simulink model "generic_IsaacV3"  (R2015a)
settings: Solver=ode3  StartTime=0.0  StopTime=inf  FixedStep=0.001  RelTol=1e-3
values from neighbouring files (symbols this model uses):
  coast_domain = 0.1    [LoadVar.m]
  DifferentialFactor = 0.5    [LoadVar.m]
  g = 9.81    [LoadVar.m]
  GearRatio = 10.364    [LoadVar.m]
  Gr = 10.32    [LoadVar.m]
  Lf = 0.78    [LoadVar.m]
  Lr = 0.745    [LoadVar.m]
  M = 265    [LoadVar.m]
  max_coast_Nm = 0    [LoadVar.m]
  MaxSteeringAngle = 24.635    [LoadVar.m]
  mu_max = 1.5    [LoadVar.m]
  ped_max_limiet = 1    [LoadVar.m]
  pedal_position_maxacc = 0.9    [LoadVar.m]
  Reff = 0.2325    [LoadVar.m]
  regen_activation_kph = 15    [LoadVar.m]
  slewbreak_domain = 0.15    [LoadVar.m]
  Sr = 0.6    [LoadVar.m]
  T_max_Nm = 40    [LoadVar.m]
  T_min_Nm = -15    [LoadVar.m]
  TireRadius = 0.4572/2    (= 0.2286)    [LoadVar.m]
  Tmax = 40    [LoadVar.m]
  TrackLength = 1.534    [LoadVar.m]
  TrackWidth = 1.200    (= 1.2)    [LoadVar.m]
libraries: CarMaker4SL x21, simulink x7
(part 1 of 3)
settings Model: ExtModeAutoUpdateStatusClock=off  Creator=fh  LastModifiedBy=Alexander
settings DataIOCC: SignalLoggingSaveFormat=ModelDataLogs  SignalLoggingName=sigsOut
settings OptimizationCC: BooleanDataType=off  ExpressionDepthLimit=2147483647  InitFltsAndDblsToZero=on
settings DebuggingCC: SaveWithParameterizedLinksMsg=none  UnderspecifiedInitializationDetection=Classic  MergeDetectMultiDrivingBlocksExec=none  SignalResolutionControl=TryResolveAllWithWarning  MultiTaskDSMMsg=warning  MultiTaskCondExecSysMsg=none  FcnCallInpInsideContextMsg=UseLocalSettings  StateNameClashWarn=warning
settings HardwareCC: TargetLongLongMode=on  TargetIntDivRoundTo=Zero  TargetEndianess=LittleEndian  TargetHWDeviceType=MATLAB Host  ProdEqTarget=off
settings CodeAppCC: MaxIdLength=63
settings GRTTargetCC: TargetFcnLib=ansi_tfl_tmw.mat  CombineOutputUpdateFcns=off  GRTInterface=on

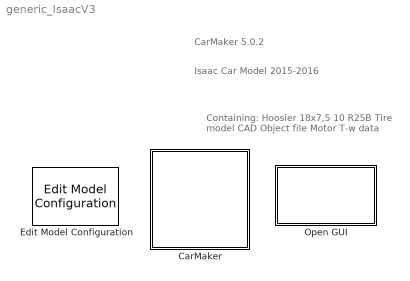
== system generic_IsaacV3 ==
  note: Isaac Car Model 2015-2016
  note: Containing:
      | Hoosier 18x7,5 10 R25B Tire model
      | CAD Object file
      | Motor T-w data
  note: CarMaker 5.0.2
  CarMaker : Subsystem  TreatAsAtomicUnit=on
      mask Display: image(imread('CarMaker4SLss.bmp'));
  Edit Model Configuration : CarMaker4SL/Edit Model Configuration
  Open GUI : Subsystem  LoadFcn=if ~length(which('cmcmd')), cmenv; end
      settings: OpenFcn=cmblockmagic('gui_fix_display'); CM_Simulink
      mask Display: image(imread('CarMakerGUI.bmp'));

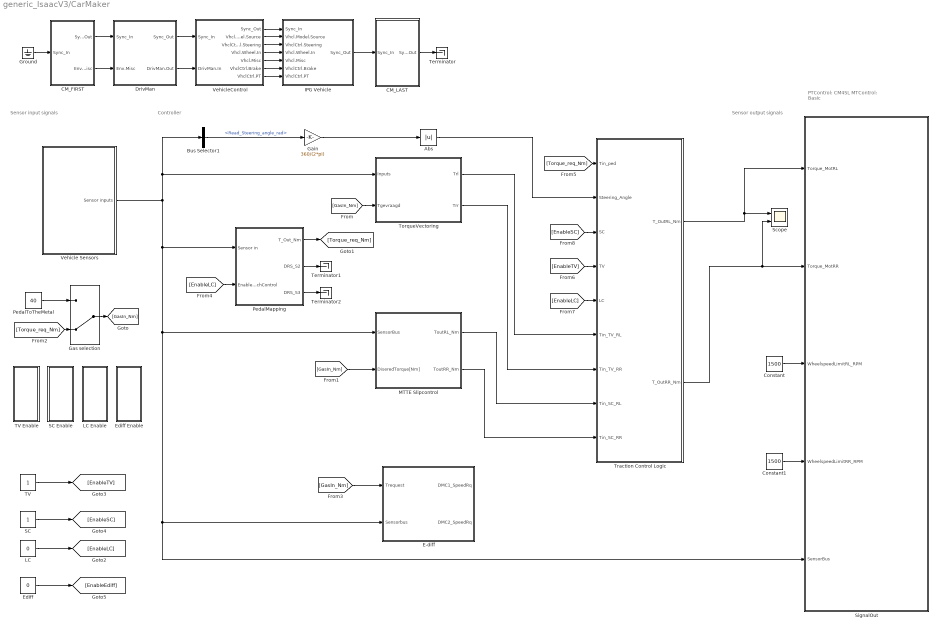
== system generic_IsaacV3/CarMaker ==
  note: PTControl: CM4SL
      | MTControl: Basic
  note: Controller
  note: Sensor output signals
  note: Sensor input signals
  Abs : Abs
  Bus Selector1 : BusSelector  OutputSignals=SensorBus.Read_Steering_angle_rad
  CM_FIRST : Subsystem
  CM_LAST : Subsystem
  Constant : Constant  Value=1500
  Constant1 : Constant  Value=1500
  DrivMan : Subsystem
  E-diff : Subsystem
  Ediff : Constant  Value=0
  Ediff Enable : Subsystem  DialogController=hmiCreateDDGDialog  IsWebBlock=on  mask(MathWorksWebBlock){webBlockId=a87a3f71-7ab5-45be-a85e-108e57319b55, webBlockType=toggleswitch, ShowInLibBrowser=on, ShowInitialText=on, HMISrcModelName=generic_IsaacV3}
      mask prompts: webBlockId "WebBlock Id"; webBlockType "WebBlock Type"; HMISrcModelName "Source Model"
      mask Help: helpview([docroot '/mapfiles/simulink.map'], 'hmi_toggle_switch')
      mask Display:
      | if strcmp(get_param(bdroot(gcb),'BlockDiagramType'), 'library')
      |     image([(matlabroot) '/toolbox/simulink/hmi/icons/ToggleSwitch.png']);
      | end
  Gain : Gain  Gain=360/(2*pi)
  Gas selection : ManualSwitch  CurrentSetting=0
  Ground : Ground
  IPG Vehicle : Subsystem  TreatAsAtomicUnit=on
  LC : Constant  Value=0
  LC Enable : Subsystem  DialogController=hmiCreateDDGDialog  IsWebBlock=on  mask(MathWorksWebBlock){webBlockId=f0719819-69bc-48b2-89e1-4e9d590658cc, webBlockType=toggleswitch, ShowInLibBrowser=on, ShowInitialText=on, HMISrcModelName=generic_IsaacV3}
      mask prompts: webBlockId "WebBlock Id"; webBlockType "WebBlock Type"; HMISrcModelName "Source Model"
      mask Help: helpview([docroot '/mapfiles/simulink.map'], 'hmi_toggle_switch')
      mask Display:
      | if strcmp(get_param(bdroot(gcb),'BlockDiagramType'), 'library')
      |     image([(matlabroot) '/toolbox/simulink/hmi/icons/ToggleSwitch.png']);
      | end
  MTTE Slipcontrol : Subsystem
  PedalMapping : Subsystem
  PedalToTheMetal : Constant  Value=40
  SC : Constant
  SC Enable : Subsystem  DialogController=hmiCreateDDGDialog  IsWebBlock=on  mask(MathWorksWebBlock){webBlockId=0a73dbf7-03b2-456b-97db-f8b49fcd234d, webBlockType=toggleswitch, ShowInLibBrowser=on, ShowInitialText=on, HMISrcModelName=generic_IsaacV3}
      mask prompts: webBlockId "WebBlock Id"; webBlockType "WebBlock Type"; HMISrcModelName "Source Model"
      mask Help: helpview([docroot '/mapfiles/simulink.map'], 'hmi_toggle_switch')
      mask Display:
      | if strcmp(get_param(bdroot(gcb),'BlockDiagramType'), 'library')
      |     image([(matlabroot) '/toolbox/simulink/hmi/icons/ToggleSwitch.png']);
      | end
  Scope : Scope  NumInputPorts=2
      settings: YMin=-20~-20  YMax=50~50  SaveName=ScopeData7
  SignalOut : Subsystem
  TV : Constant
  TV Enable : Subsystem  DialogController=hmiCreateDDGDialog  IsWebBlock=on  mask(MathWorksWebBlock){webBlockId=11ac5f76-cd76-4bde-b9bd-54c96ed035c7, webBlockType=toggleswitch, ShowInLibBrowser=on, ShowInitialText=on, HMISrcModelName=generic_IsaacV3}
      mask prompts: webBlockId "WebBlock Id"; webBlockType "WebBlock Type"; HMISrcModelName "Source Model"
      mask Help: helpview([docroot '/mapfiles/simulink.map'], 'hmi_toggle_switch')
      mask Display:
      | if strcmp(get_param(bdroot(gcb),'BlockDiagramType'), 'library')
      |     image([(matlabroot) '/toolbox/simulink/hmi/icons/ToggleSwitch.png']);
      | end
  Terminator : Terminator
  Terminator1 : Terminator
  Terminator2 : Terminator
  TorqueVectoring : Subsystem
  Traction Control Logic : Stateflow chart  TreatAsAtomicUnit=on
  Vehicle Sensors : Subsystem
  VehicleControl : Subsystem
  wires:
  DrivMan/2(DrivMan.Out) -> VehicleControl/2(DrivMan.In)
  DrivMan/1(Sync_Out) -> VehicleControl/1(Sync_In)
  CM_FIRST/2(Env.Misc) -> DrivMan/2(Env.Misc)
  CM_FIRST/1(Sync_Out) -> DrivMan/1(Sync_In)
  CM_LAST/1(Sync_Out) -> Terminator/1
  IPG Vehicle/1(Sync_Out) -> CM_LAST/1(Sync_In)
  VehicleControl/1(Sync_Out) -> IPG Vehicle/1(Sync_In)
  VehicleControl/3(VhclCtrl.Steering) -> IPG Vehicle/3(VhclCtrl.Steering)
  VehicleControl/4(Vhcl.Wheel.In) -> IPG Vehicle/4(Vhcl.Wheel.In)
  VehicleControl/5(Vhcl.Misc) -> IPG Vehicle/5(Vhcl.Misc)
  VehicleControl/6(VhclCtrl.Brake) -> IPG Vehicle/6(VhclCtrl.Brake)
  VehicleControl/7(VhclCtrl.PT) -> IPG Vehicle/7(VhclCtrl.PT)
  VehicleControl/2(Vhcl.Model.Source) -> IPG Vehicle/2(Vhcl.Model.Source)
  Ground/1 -> CM_FIRST/1(Sync_In)
  Vehicle Sensors/1(Sensor inputs) -> SignalOut/5(SensorBus), E-diff/2(Sensorbus), MTTE Slipcontrol/1(SensorBus), PedalMapping/1(Sensor in), Bus Selector1/1, TorqueVectoring/1(Inputs)
  PedalToTheMetal/1 -> Gas selection/1
  Gas selection/1 -> [GasIn_Nm]
  [GasIn_Nm] -> TorqueVectoring/2(Tgevraagd)
  [GasIn_Nm] -> MTTE Slipcontrol/2(DiseredTorque[Nm])
  PedalMapping/1(T_Out_Nm) -> [Torque_req_Nm]
  [Torque_req_Nm] -> Gas selection/2
  [GasIn_Nm] -> E-diff/1(Trequest)
  Constant/1 -> SignalOut/3(WheelspeedLimitRL_RPM)
  Constant1/1 -> SignalOut/4(WheelspeedLimitRR_RPM)
  [EnableLC] -> PedalMapping/2(EnableLaunchControl)
  LC/1 -> [EnableLC]
  TV/1 -> [EnableTV]
  SC/1 -> [EnableSC]
  Ediff/1 -> [EnableEdiff]
  Bus Selector1/1 -> Gain/1  "<Read_Steering_angle_rad>"
  Gain/1 -> Abs/1
  [Torque_req_Nm] -> Traction Control Logic/1(Tin_ped)
  [EnableTV] -> Traction Control Logic/4(TV)
  [EnableLC] -> Traction Control Logic/5(LC)
  [EnableSC] -> Traction Control Logic/3(SC)
  TorqueVectoring/1(Trl) -> Traction Control Logic/6(Tin_TV_RL)
  MTTE Slipcontrol/1(ToutRL_Nm) -> Traction Control Logic/8(Tin_SC_RL)
  TorqueVectoring/2(Trr) -> Traction Control Logic/7(Tin_TV_RR)
  MTTE Slipcontrol/2(ToutRR_Nm) -> Traction Control Logic/9(Tin_SC_RR)
  Traction Control Logic/1(T_OutRL_Nm) -> Scope/1, SignalOut/1(Torque_MotRL)
  Traction Control Logic/2(T_OutRR_Nm) -> Scope/2, SignalOut/2(Torque_MotRR)
  Abs/1 -> Traction Control Logic/2(Steering_Angle)
  PedalMapping/2(DRS_S2) -> Terminator1/1
  PedalMapping/3(DRS_S3) -> Terminator2/1

== system generic_IsaacV3/Open GUI ==
  S-Function : S-Function  FunctionName=cm_gui

== system generic_IsaacV3/CarMaker/CM_FIRST ==
  Sync_In : Inport
  Bus Creator1 : BusCreator  Inputs=9
  Demux : Demux  Outputs=9
  Environment : S-Function  FunctionName=CM_Sfun  Parameters='Environment'
  IoIn : S-Function  FunctionName=CM_Sfun  Parameters='IoIn'
  Sync_Out : Outport
  Env.Misc : Outport  Port=2
  wires:
  Bus Creator1/1 -> Env.Misc/1
  Environment/2 -> Demux/1
  Demux/4 -> Bus Creator1/4  "Env AirHumidity"
  Demux/3 -> Bus Creator1/3  "Env AirPressure"
  Demux/2 -> Bus Creator1/2  "Env AirDensity"
  Demux/1 -> Bus Creator1/1  "Env Temperature"
  Environment/1 -> Sync_Out/1
  IoIn/1 -> Environment/1
  Sync_In/1 -> IoIn/1
  Demux/5 -> Bus Creator1/5  "Env Time"
  Demux/6 -> Bus Creator1/6  "Env SolarRadiation"
  Demux/7 -> Bus Creator1/7  "Env WindVel_tot x"
  Demux/8 -> Bus Creator1/8  "Env WindVel_tot y"
  Demux/9 -> Bus Creator1/9  "Env WindVel_tot z"

== system generic_IsaacV3/CarMaker/CM_LAST ==
  Sync_In : Inport
  CM_User : S-Function  FunctionName=CM_Sfun  Parameters='CM_User'
  IoOut : S-Function  FunctionName=CM_Sfun  Parameters='IoOut'
  Sync_Out : Outport
  wires:
  IoOut/1 -> Sync_Out/1
  CM_User/1 -> IoOut/1
  Sync_In/1 -> CM_User/1

== system generic_IsaacV3/CarMaker/DrivMan ==
  note: There's rarely a reason to override DrivMan signals.
      | Use the VehicleControl interface for this purpose.
  Sync_In : Inport
  Env.Misc : Inport  Port=2
  BusCreator : BusCreator  Inputs=17
  Demux : Demux  Outputs=17
  DrivMan : S-Function  FunctionName=CM_Sfun  Parameters='DrivMan'
  Sync_Out : Outport
  DrivMan.Out : Outport  Port=2
  wires:
  Demux/17 -> BusCreator/17  "DrivMan Steering Trq"
  Demux/16 -> BusCreator/16  "DrivMan Steering AngAcc"
  Demux/15 -> BusCreator/15  "DrivMan Steering AngVel"
  Demux/14 -> BusCreator/14  "DrivMan Steering Ang"
  Demux/13 -> BusCreator/13  "DrivMan Gas"
  Demux/12 -> BusCreator/12  "DrivMan Clutch"
  Demux/11 -> BusCreator/11  "DrivMan BrakePark"
  Demux/10 -> BusCreator/10  "DrivMan Brake"
  Demux/9 -> BusCreator/9  "DrivMan GearNo"
  Demux/8 -> BusCreator/8  "DrivMan SelectorCtrl"
  Demux/7 -> BusCreator/7  "DrivMan UserSignal4"
  Demux/6 -> BusCreator/6  "DrivMan UserSignal3"
  Demux/5 -> BusCreator/5  "DrivMan UserSignal2"
  Demux/4 -> BusCreator/4  "DrivMan UserSignal1"
  Demux/3 -> BusCreator/3  "DrivMan UserSignal0"
  Demux/2 -> BusCreator/2  "DrivMan Key"
  Demux/1 -> BusCreator/1  "DrivMan SST"
  Env.Misc/1 -> DrivMan/2
  Sync_In/1 -> DrivMan/1
  DrivMan/1 -> Sync_Out/1
  BusCreator/1 -> DrivMan.Out/1
  DrivMan/2 -> Demux/1

== system generic_IsaacV3/CarMaker/E-diff ==
  Trequest : Inport
  Sensorbus : Inport  Port=2
  Bus Selector1 : BusSelector  OutputSignals=Vehicle_velocity_mps,SensorBus.Read_Steering_angle_rad
  Constant : Constant
  Constant1 : Constant  Value=0
  Constant2 : Constant  Value=0
  Differential_Statemachine : Stateflow chart  TreatAsAtomicUnit=on
  E-Differential : Subsystem
  Gain : Gain  Gain=180/pi
  Logical Operator1 : Logic  Operator=OR  AllPortsSameDT=off  OutDataTypeStr=boolean
  Memory : Memory  X0=zeros(10,1)  InheritSampleTime=on
  Memory1 : Memory  X0=zeros(10,1)  InheritSampleTime=on
  ThrottleStatus : MATLAB Function  TreatAsAtomicUnit=on
  VelocityStatus : MATLAB Function  TreatAsAtomicUnit=on
  DMC1_SpeedRq : Outport
  DMC2_SpeedRq : Outport  Port=2
  wires:
  Trequest/1 -> ThrottleStatus/1(CurrentTorqueRequest)
  VelocityStatus/2(ArrayNext) -> Memory1/1
  Memory1/1 -> VelocityStatus/2(ArrayPrevious)
  Gain/1 -> Differential_Statemachine/2(SteeringAngle), E-Differential/3(SteeringAngle)
  Differential_Statemachine/1(DMC1_SpeedRq) -> DMC1_SpeedRq/1
  ThrottleStatus/1(Accelerating) -> Logical Operator1/1
  Constant/1 -> Differential_Statemachine/1(EnableDifferential)
  ThrottleStatus/2(ArrayNext) -> Memory/1
  E-Differential/1(DMC1_SpeedRq) -> Differential_Statemachine/5(SpeedRq1)
  Logical Operator1/1 -> E-Differential/1(Accelerating)
  E-Differential/2(DMC2_SpeedRq) -> Differential_Statemachine/6(SpeedRq2)
  VelocityStatus/1(Accelerating) -> Logical Operator1/2
  Memory/1 -> ThrottleStatus/2(ArrayPrevious)
  Differential_Statemachine/2(DMC2_SpeedRq) -> DMC2_SpeedRq/1
  Sensorbus/1 -> Bus Selector1/1
  Bus Selector1/2 -> Gain/1  "<Read_Steering_angle_rad>"
  Bus Selector1/1 -> VelocityStatus/1(CurrentVelocity), E-Differential/2(Velocity)  "<Vehicle_velocity_mps>"
  Constant1/1 -> Differential_Statemachine/3(WheelSpeedError)
  Constant2/1 -> Differential_Statemachine/4(SteeringAngleError)

== system generic_IsaacV3/CarMaker/Ediff Enable ==

== system generic_IsaacV3/CarMaker/IPG Vehicle ==
  Sync_In : Inport
  Vhcl.Model.Source : Inport  Port=2
  VhclCtrl.Steering : Inport  Port=3
  Vhcl.Wheel.In : Inport  Port=4
  Vhcl.Misc : Inport  Port=5
  VhclCtrl.Brake : Inport  Port=6
  VhclCtrl.PT : Inport  Port=7
  Brake : Subsystem
  CarAndTrailer : Subsystem
  PowerTrain : Subsystem
  Stop Simulation : Stop
  VehicleSource_BuiltIn : simulink/Logic and Bit Operations/Compare To Constant  relop=~=  const=1  OutDataTypeStr=boolean  ZeroCross=off
  Sync_Out : Outport
  wires:
  VhclCtrl.PT/1 -> PowerTrain/3(VhclCtrl.PT)
  Brake/1(Sync_Out) -> PowerTrain/1(Sync_In)
  CarAndTrailer/1(Sync_Out) -> Brake/1(Sync_In)
  CarAndTrailer/2(Brake.IF.In) -> Brake/2(Brake.IF.In)
  VhclCtrl.Brake/1 -> Brake/3(VhclCtrl.Brake)
  PowerTrain/1(Sync_Out) -> Sync_Out/1
  Vhcl.Misc/1 -> CarAndTrailer/4(Vhcl.Misc)
  Vhcl.Wheel.In/1 -> CarAndTrailer/3(Vhcl.Wheel.In)
  VhclCtrl.Steering/1 -> CarAndTrailer/2(VhclCtrl.Steering)
  Sync_In/1 -> CarAndTrailer/1(Sync_In)
  Vhcl.Model.Source/1 -> VehicleSource_BuiltIn/1
  VehicleSource_BuiltIn/1 -> Stop Simulation/1
  Brake/2(Vhcl.Wheel.PT) -> PowerTrain/2(Vhcl.Wheel.PT)

== system generic_IsaacV3/CarMaker/LC Enable ==

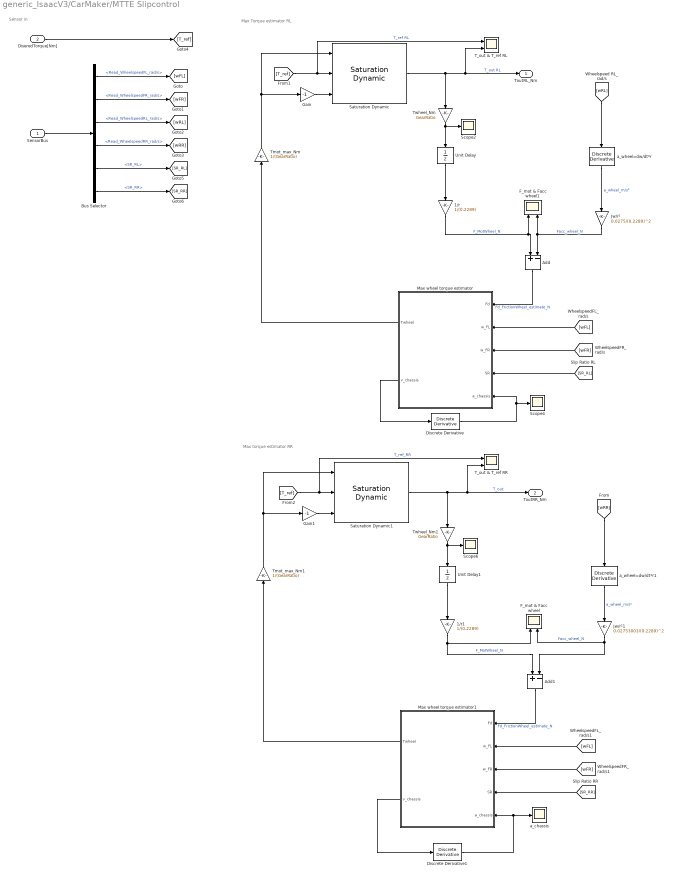
== system generic_IsaacV3/CarMaker/MTTE Slipcontrol ==
  note: Max torque estimator RR
  note: Max Torque estimator RL
  note: Sensor in
  SensorBus : Inport
  DiseredTorque[Nm] : Inport  Port=2
  1/r : Gain  Gain=1/(0.2289)
  1/r1 : Gain  Gain=1/(0.2289)
  Add : Sum  Inputs=+|-
  Add1 : Sum  Inputs=+|-
  Bus Selector : BusSelector  OutputSignals=SensorBus.Read_WheelspeedFL_rad/s,SensorBus.Read_WheelspeedFR_rad/s,SensorBus.Read_WheelspeedRL_rad/s,SensorBus.Read_WheelspeedRR_rad/s,SR_RL,SR_RR
  Discrete Derivative : simulink/Discrete/Discrete Derivative  gainval=1.0  ICPrevScaledInput=0.0  InputProcessing=Inherited  OutMin=[]  OutMax=[]  OutDataType=fixdt(1, 16)  OutScaling=2^-10  DoSatur=off
  Discrete Derivative1 : simulink/Discrete/Discrete Derivative  gainval=1.0  ICPrevScaledInput=0.0  InputProcessing=Inherited  OutMin=[]  OutMax=[]  OutDataType=fixdt(1, 16)  OutScaling=2^-10  DoSatur=off
  F_mot & Facc wheel : Scope  NumInputPorts=2
      settings: YMin=-300~-1755  YMax=600~1755  SaveName=ScopeData23
  F_mot & Facc wheel1 : Scope  NumInputPorts=2
      settings: YMin=250~10  YMax=1750~22  SaveName=ScopeData18
  Gain : Gain  Gain=-1
  Gain1 : Gain  Gain=-1
  Jw/r² : Gain  Gain=0.0275/(0.2289)^2
  Jw/r²1 : Gain  Gain=0.02753003/(0.2289)^2
  Max wheel torque estimator : MATLAB Function  TreatAsAtomicUnit=on
  Max wheel torque estimator1 : MATLAB Function  TreatAsAtomicUnit=on
  Saturation Dynamic : simulink/Discontinuities/Saturation Dynamic  OutMin=[]  OutMax=[]  OutDataTypeStr=Inherit: Same as second input  OutDataType=fixdt(1, 16)  OutScaling=2^-10  DoSatur=off
  Saturation Dynamic1 : simulink/Discontinuities/Saturation Dynamic  OutMin=[]  OutMax=[]  OutDataTypeStr=Inherit: Same as second input  OutDataType=fixdt(1, 16)  OutScaling=2^-10  DoSatur=off
  Scope2 : Scope
      settings: SaveName=ScopeData22
  Scope4 : Scope
      settings: YMin=-10  YMax=10  SaveName=ScopeData24
  Scope6 : Scope
      settings: SaveName=ScopeData26
  T_out & T_ref RL : Scope  NumInputPorts=2
      settings: YMin=-50~-50  YMax=50~50  SaveName=ScopeData17
  T_out & T_ref RR : Scope  NumInputPorts=2
      settings: YMin=-50~-50  YMax=50~50  SaveName=ScopeData28
  Tmot_max_Nm : Gain  Gain=1/(GearRatio)
  Tmot_max_Nm1 : Gain  Gain=1/(GearRatio)
  Twheel_Nm : Gain  Gain=GearRatio
  Twheel_Nm1 : Gain  Gain=GearRatio
  Unit Delay : UnitDelay  SampleTime=-1
  Unit Delay1 : UnitDelay  SampleTime=-1
  a_chassis : Scope
      settings: YMin=-10  YMax=10  SaveName=ScopeData27
  a_wheel=dw/dt*r : simulink/Discrete/Discrete Derivative  gainval=0.2289  ICPrevScaledInput=0.0  InputProcessing=Inherited  OutMin=[]  OutMax=[]  OutDataType=fixdt(1, 16)  OutScaling=2^-10  DoSatur=off
  a_wheel=dw/dt*r1 : simulink/Discrete/Discrete Derivative  gainval=0.2289  ICPrevScaledInput=0.0  InputProcessing=Inherited  OutMin=[]  OutMax=[]  OutDataType=fixdt(1, 16)  OutScaling=2^-10  DoSatur=off
  ToutRL_Nm : Outport
  ToutRR_Nm : Outport  Port=2
  wires:
  Unit Delay/1 -> 1/r/1
  a_wheel=dw/dt*r/1 -> Jw/r²/1  "a_wheel_m/s²"
  1/r/1 -> F_mot & Facc wheel1/1, Add/1  "F_MotWheel_N"
  Jw/r²/1 -> Add/2, F_mot & Facc wheel1/2  "Facc_wheel_N"
  Add/1 -> Max wheel torque estimator/1(Fd)  "Fd_FrictionWheel_estimate_N"
  Max wheel torque estimator/1(Twheel) -> Tmot_max_Nm/1
  [wFL] -> Max wheel torque estimator/2(w_FL)
  [wFR] -> Max wheel torque estimator/3(w_FR)
  Saturation Dynamic/1 -> Twheel_Nm/1, ToutRL_Nm/1, T_out & T_ref RL/2  "T_out RL"
  [T_ref] -> Saturation Dynamic/2, T_out & T_ref RL/1  "T_ref RL"
  Max wheel torque estimator/2(v_chassis) -> Discrete Derivative/1
  Discrete Derivative/1 -> Max wheel torque estimator/5(a_chassis), Scope4/1
  SensorBus/1 -> Bus Selector/1
  Bus Selector/1 -> [wFL]  "<Read_WheelspeedFL_rad/s>"
  Bus Selector/2 -> [wFR]  "<Read_WheelspeedFR_rad/s>"
  Bus Selector/3 -> [wRL]  "<Read_WheelspeedRL_rad/s>"
  [wRL] -> a_wheel=dw/dt*r/1
  Twheel_Nm/1 -> Scope2/1, Unit Delay/1
  Gain/1 -> Saturation Dynamic/3
  Tmot_max_Nm/1 -> Gain/1, Saturation Dynamic/1
  Unit Delay1/1 -> 1/r1/1
  a_wheel=dw/dt*r1/1 -> Jw/r²1/1  "a_wheel_m/s²"
  1/r1/1 -> F_mot & Facc wheel/1, Add1/1  "F_MotWheel_N"
  Jw/r²1/1 -> Add1/2, F_mot & Facc wheel/2  "Facc_wheel_N"
  Add1/1 -> Max wheel torque estimator1/1(Fd)  "Fd_FrictionWheel_estimate_N"
  Max wheel torque estimator1/1(Twheel) -> Tmot_max_Nm1/1
  Saturation Dynamic1/1 -> Twheel_Nm1/1, ToutRR_Nm/1, T_out & T_ref RR/2  "T_out"
  [T_ref] -> Saturation Dynamic1/2, T_out & T_ref RR/1  "T_ref_RR"
  Max wheel torque estimator1/2(v_chassis) -> Discrete Derivative1/1
  [wRR] -> a_wheel=dw/dt*r1/1
  Twheel_Nm1/1 -> Scope6/1, Unit Delay1/1
  Gain1/1 -> Saturation Dynamic1/3
  Tmot_max_Nm1/1 -> Gain1/1, Saturation Dynamic1/1
  Bus Selector/4 -> [wRR]  "<Read_WheelspeedRR_rad/s>"
  DiseredTorque[Nm]/1 -> [T_ref]
  Bus Selector/5 -> [SR_RL]  "<SR_RL>"
  Bus Selector/6 -> [SR_RR]  "<SR_RR>"
  [SR_RL] -> Max wheel torque estimator/4(SR)
  Discrete Derivative1/1 -> a_chassis/1, Max wheel torque estimator1/5(a_chassis)
  [wFL] -> Max wheel torque estimator1/2(w_FL)
  [wFR] -> Max wheel torque estimator1/3(w_FR)
  [SR_RR] -> Max wheel torque estimator1/4(SR)

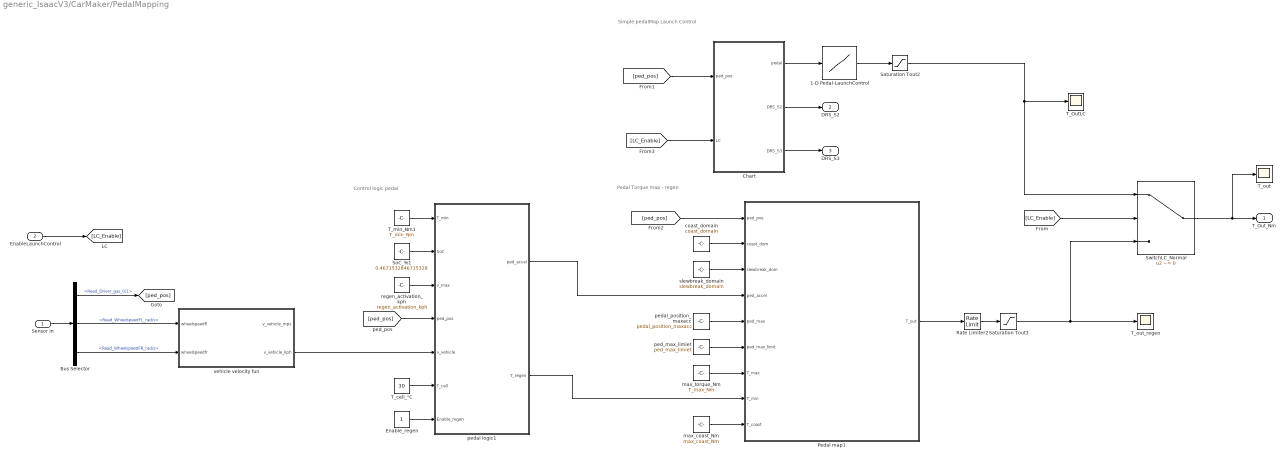
== system generic_IsaacV3/CarMaker/PedalMapping ==
  note: Simple pedalMap Launch Control
  note: Pedal Torque map - regen
  note: Control logic pedal
  Sensor in : Inport
  EnableLaunchControl : Inport  Port=2
  1-D Pedal-LaunchControl : Lookup_n-D  NumberOfTableDimensions=1  BreakpointsForDimension1=[0,0.1,0.8,1]  Table=[0,0,T_max_Nm,T_max_Nm]  InternalRulePriority=Speed  RndMeth=Simplest  InputSameDT=on
  Bus Selector : BusSelector  OutputSignals=SensorBus.Read_Driver_gas_0/1,SensorBus.Read_WheelspeedFL_rad/s,SensorBus.Read_WheelspeedFR_rad/s
  Chart : Stateflow chart  TreatAsAtomicUnit=on
  Enable_regen : Constant
  Pedal map1 : MATLAB Function  TreatAsAtomicUnit=on
  Rate Limiter2 : RateLimiter  RisingSlewLimit=2000  FallingSlewLimit=-2000  SampleTimeMode=inherited
  Saturation Tout2 : Saturate  UpperLimit=T_max_Nm  LowerLimit=0
  Saturation Tout3 : Saturate  UpperLimit=40  LowerLimit=-40
  SoC_%1 : Constant  Value=0.4671532846715328
  SwitchLC_Normal : Switch  Criteria=u2 ~= 0
  T_OutLC : Scope
      settings: YMin=-50  YMax=50  SaveName=ScopeData8
  T_cell_°C : Constant  Value=30
  T_min_Nm1 : Constant  Value=T_min_Nm
  T_out : Scope
      settings: YMin=-50  YMax=50  SaveName=ScopeData10
  T_out_regen : Scope
      settings: YMin=-50  YMax=50
  coast_domain : Constant  Value=coast_domain
  max_coast_Nm : Constant  Value=max_coast_Nm
  max_torque_Nm : Constant  Value=T_max_Nm
  ped_max_limiet : Constant  Value=ped_max_limiet
  pedal logic1 : Stateflow chart  TreatAsAtomicUnit=on
  pedal_position_maxacc : Constant  Value=pedal_position_maxacc
  regen_activation_kph : Constant  Value=regen_activation_kph
  slewbreak_domain : Constant  Value=slewbreak_domain
  vehicle velocity fun : MATLAB Function  TreatAsAtomicUnit=on
  T_Out_Nm : Outport
  DRS_S2 : Outport  Port=2
  DRS_S3 : Outport  Port=3
  wires:
  Sensor in/1 -> Bus Selector/1
  Bus Selector/2 -> vehicle velocity fun/1(wheelspeedfl)  "<Read_WheelspeedFL_rad/s>"
  Bus Selector/3 -> vehicle velocity fun/2(wheelspeedfr)  "<Read_WheelspeedFR_rad/s>"
  Bus Selector/1 -> [ped_pos]  "<Read_Driver_gas_0/1>"
  Saturation Tout2/1 -> T_OutLC/1, SwitchLC_Normal/1
  1-D Pedal-LaunchControl/1 -> Saturation Tout2/1
  SwitchLC_Normal/1 -> T_out/1, T_Out_Nm/1
  [LC_Enable] -> SwitchLC_Normal/2
  Rate Limiter2/1 -> Saturation Tout3/1
  coast_domain/1 -> Pedal map1/2(coast_dom)
  T_min_Nm1/1 -> pedal logic1/1(T_min)
  pedal_position_maxacc/1 -> Pedal map1/5(ped_max)
  slewbreak_domain/1 -> Pedal map1/3(slewbreak_dom)
  Saturation Tout3/1 -> SwitchLC_Normal/3, T_out_regen/1
  [ped_pos] -> Pedal map1/1(ped_pos)
  T_cell_°C/1 -> pedal logic1/6(T_cell)
  SoC_%1/1 -> pedal logic1/2(SoC)
  ped_max_limiet/1 -> Pedal map1/6(ped_max_limit)
  pedal logic1/2(T_regen) -> Pedal map1/8(T_min)
  max_coast_Nm/1 -> Pedal map1/9(T_coast)
  regen_activation_kph/1 -> pedal logic1/3(v_max)
  Enable_regen/1 -> pedal logic1/7(Enable_regen)
  pedal logic1/1(ped_accel) -> Pedal map1/4(ped_accel)
  [ped_pos] -> pedal logic1/4(ped_pos)
  max_torque_Nm/1 -> Pedal map1/7(T_max)
  Pedal map1/1(T_out) -> Rate Limiter2/1
  vehicle velocity fun/2(v_vehicle_kph) -> pedal logic1/5(v_vehicle)
  Chart/1(pedal) -> 1-D Pedal-LaunchControl/1
  [ped_pos] -> Chart/1(ped_pos)
  EnableLaunchControl/1 -> [LC_Enable]
  [LC_Enable] -> Chart/2(LC)
  Chart/2(DRS_S2) -> DRS_S2/1
  Chart/3(DRS_S3) -> DRS_S3/1

== system generic_IsaacV3/CarMaker/SC Enable ==

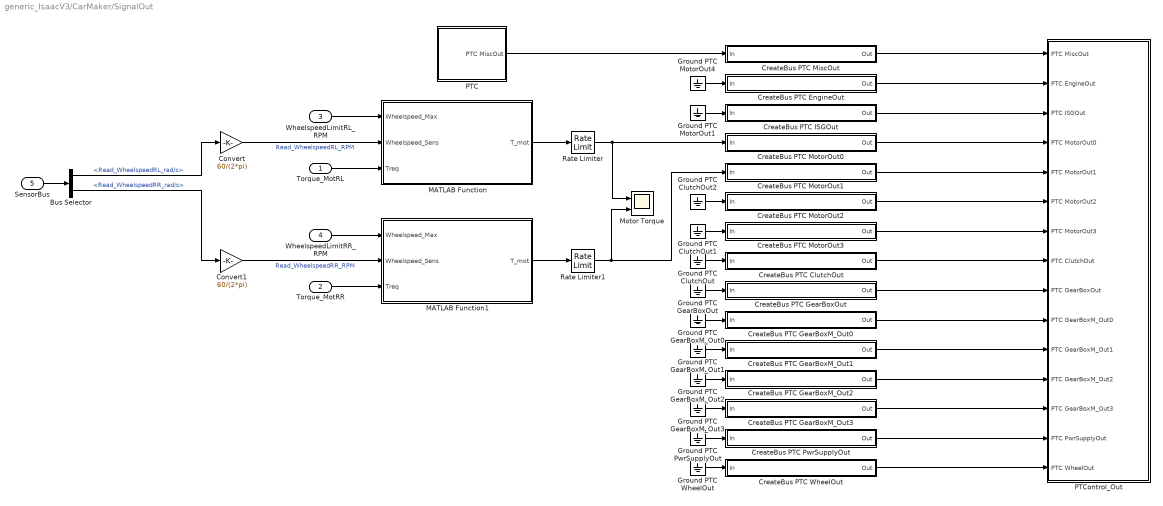
== system generic_IsaacV3/CarMaker/SignalOut ==
  Torque_MotRL : Inport
  Torque_MotRR : Inport  Port=2
  WheelspeedLimitRL_RPM : Inport  Port=3
  WheelspeedLimitRR_RPM : Inport  Port=4
  SensorBus : Inport  Port=5
  Bus Selector : BusSelector  OutputSignals=SensorBus.Read_WheelspeedRL_rad/s,SensorBus.Read_WheelspeedRR_rad/s
  Convert : Gain  Gain=60/(2*pi)
  Convert1 : Gain  Gain=60/(2*pi)
  CreateBus PTC ClutchOut : Subsystem
  CreateBus PTC EngineOut : Subsystem
  CreateBus PTC GearBoxM_Out0 : Subsystem
  CreateBus PTC GearBoxM_Out1 : Subsystem
  CreateBus PTC GearBoxM_Out2 : Subsystem
  CreateBus PTC GearBoxM_Out3 : Subsystem
  CreateBus PTC GearBoxOut : Subsystem
  CreateBus PTC ISGOut : Subsystem
  CreateBus PTC MiscOut : Subsystem
  CreateBus PTC MotorOut0 : Subsystem
  CreateBus PTC MotorOut1 : Subsystem
  CreateBus PTC MotorOut2 : Subsystem
  CreateBus PTC MotorOut3 : Subsystem
  CreateBus PTC PwrSupplyOut : Subsystem
  CreateBus PTC WheelOut : Subsystem
  Ground PTC ClutchOut : Ground
  Ground PTC ClutchOut1 : Ground
  Ground PTC ClutchOut2 : Ground
  Ground PTC GearBoxM_Out{0..3} (4 alike) : Ground
  Ground PTC GearBoxOut : Ground
  Ground PTC MotorOut1 : Ground
  Ground PTC MotorOut4 : Ground
  Ground PTC PwrSupplyOut : Ground
  Ground PTC WheelOut : Ground
  MATLAB Function : MATLAB Function  TreatAsAtomicUnit=on
  MATLAB Function1 : MATLAB Function  TreatAsAtomicUnit=on
  Motor Torque : Scope  NumInputPorts=2
      settings: YMin=0~0  YMax=0.5~0.5  SaveName=ScopeData13
  PTC : Subsystem
  PTControl_Out : Subsystem
  Rate Limiter : RateLimiter  RisingSlewLimit=1000  FallingSlewLimit=-1000
  Rate Limiter1 : RateLimiter  RisingSlewLimit=1000  FallingSlewLimit=-1000
  wires:
  Ground PTC GearBoxM_Out1/1 -> CreateBus PTC GearBoxM_Out1/1(In)
  CreateBus PTC MotorOut2/1(Out) -> PTControl_Out/6(PTC MotorOut2)
  Ground PTC GearBoxOut/1 -> CreateBus PTC GearBoxOut/1(In)
  CreateBus PTC GearBoxM_Out0/1(Out) -> PTControl_Out/10(PTC GearBoxM_Out0)
  Ground PTC GearBoxM_Out0/1 -> CreateBus PTC GearBoxM_Out0/1(In)
  Ground PTC ClutchOut/1 -> CreateBus PTC ClutchOut/1(In)
  Ground PTC MotorOut4/1 -> CreateBus PTC EngineOut/1(In)
  CreateBus PTC GearBoxM_Out3/1(Out) -> PTControl_Out/13(PTC GearBoxM_Out3)
  CreateBus PTC GearBoxM_Out1/1(Out) -> PTControl_Out/11(PTC GearBoxM_Out1)
  Ground PTC GearBoxM_Out3/1 -> CreateBus PTC GearBoxM_Out3/1(In)
  Ground PTC MotorOut1/1 -> CreateBus PTC ISGOut/1(In)
  Ground PTC PwrSupplyOut/1 -> CreateBus PTC PwrSupplyOut/1(In)
  CreateBus PTC PwrSupplyOut/1(Out) -> PTControl_Out/14(PTC PwrSupplyOut)
  Ground PTC WheelOut/1 -> CreateBus PTC WheelOut/1(In)
  CreateBus PTC WheelOut/1(Out) -> PTControl_Out/15(PTC WheelOut)
  CreateBus PTC MotorOut3/1(Out) -> PTControl_Out/7(PTC MotorOut3)
  CreateBus PTC ISGOut/1(Out) -> PTControl_Out/3(PTC ISGOut)
  CreateBus PTC MotorOut1/1(Out) -> PTControl_Out/5(PTC MotorOut1)
  CreateBus PTC GearBoxM_Out2/1(Out) -> PTControl_Out/12(PTC GearBoxM_Out2)
  CreateBus PTC ClutchOut/1(Out) -> PTControl_Out/8(PTC ClutchOut)
  Ground PTC GearBoxM_Out2/1 -> CreateBus PTC GearBoxM_Out2/1(In)
  CreateBus PTC GearBoxOut/1(Out) -> PTControl_Out/9(PTC GearBoxOut)
  CreateBus PTC EngineOut/1(Out) -> PTControl_Out/2(PTC EngineOut)
  CreateBus PTC MotorOut0/1(Out) -> PTControl_Out/4(PTC MotorOut0)
  CreateBus PTC MiscOut/1(Out) -> PTControl_Out/1(PTC MiscOut)
  PTC/1(PTC MiscOut) -> CreateBus PTC MiscOut/1(In)
  Ground PTC ClutchOut1/1 -> CreateBus PTC MotorOut3/1(In)
  Ground PTC ClutchOut2/1 -> CreateBus PTC MotorOut2/1(In)
  Torque_MotRR/1 -> MATLAB Function1/3(Treq)
  Torque_MotRL/1 -> MATLAB Function/3(Treq)
  MATLAB Function/1(T_mot) -> Rate Limiter/1
  MATLAB Function1/1(T_mot) -> Rate Limiter1/1
  WheelspeedLimitRL_RPM/1 -> MATLAB Function/1(Wheelspeed_Max)
  WheelspeedLimitRR_RPM/1 -> MATLAB Function1/1(Wheelspeed_Max)
  SensorBus/1 -> Bus Selector/1
  Bus Selector/1 -> Convert/1  "<Read_WheelspeedRL_rad/s>"
  Convert/1 -> MATLAB Function/2(Wheelspeed_Sens)  "Read_WheelspeedRL_RPM"
  Bus Selector/2 -> Convert1/1  "<Read_WheelspeedRR_rad/s>"
  Convert1/1 -> MATLAB Function1/2(Wheelspeed_Sens)  "Read_WheelspeedRR_RPM"
  Rate Limiter/1 -> CreateBus PTC MotorOut0/1(In), Motor Torque/1
  Rate Limiter1/1 -> Motor Torque/2, CreateBus PTC MotorOut1/1(In)

== system generic_IsaacV3/CarMaker/TV Enable ==

== system generic_IsaacV3/CarMaker/TorqueVectoring ==
  Inputs : Inport
  Tgevraagd : Inport  Port=2
  2-D Lookup Table1 : Lookup_n-D  BreakpointsForDimension1=[-15,-14,-13,-12,-11,-10,-9,-8,-7,-6,-5,-4,-3,-2,-1,0,1,2,3,4,5,6,7,8,9,10,11,12,13,14,15]  BreakpointsForDimension2=[200,425,650,875,1100]  Table=reshape([-510,-510,-510,-510,-500,-500,-460,-460,-460,-420,-420,-380,-340,-270,-150,0,150,270,340,380,420,420,460,460,460,500,500,500,500,500,500,-1020,-1020,-1020,-1020,-1000,-1000,-1000,-960,-960,-920,-880,-800,-690,-540,-350,0,350,540,690,800,880,920,960,960,1000,1000,1000,1020,1020,1020,1020,-1540,-1540,-1540,-1540,-1500,-1500,-1500,-1460,-1420,-1360,-1300,-1230,-1040,-800,-500,0,500,800,1040,1230,1300,1360,1420,1460,1500,1500,1500,1540,1540,1540,1540,-2020,-2020,-2020,-2020,-1980,-1960,-1920,-1920,-1860,-1790,-1690,-1540,-1330,-960,-580,0,580,960,1330,1540,1690,1790,1860,1920,1920,1960,1980,2020,2020,2020,2020,-2500,-2500,-2500,-2440,-2420,-2420,-2380,-2300,-2250,-2180,-2000,-1800,-1540,-1150,-690,0,690,1150,1540,1800,2000,2180,2250,2300,2380,2420,2420,2440,2500,2500,2500],31,5)  InternalRulePriority=Speed  RndMeth=Simplest  InputSameDT=on
  2-D Lookup Table2 : Lookup_n-D  BreakpointsForDimension1=[-15,-14,-13,-12,-11,-10,-9,-8,-7,-6,-5,-4,-3,-2,-1,0,1,2,3,4,5,6,7,8,9,10,11,12,13,14,15]  BreakpointsForDimension2=[200,425,650,875,1100]  Table=reshape([-510,-510,-510,-510,-500,-500,-460,-460,-460,-420,-420,-380,-340,-270,-150,0,150,270,340,380,420,420,460,460,460,500,500,500,500,500,500,-1020,-1020,-1020,-1020,-1000,-1000,-1000,-960,-960,-920,-880,-800,-690,-540,-350,0,350,540,690,800,880,920,960,960,1000,1000,1000,1020,1020,1020,1020,-1540,-1540,-1540,-1540,-1500,-1500,-1500,-1460,-1420,-1360,-1300,-1230,-1040,-800,-500,0,500,800,1040,1230,1300,1360,1420,1460,1500,1500,1500,1540,1540,1540,1540,-2020,-2020,-2020,-2020,-1980,-1960,-1920,-1920,-1860,-1790,-1690,-1540,-1330,-960,-580,0,580,960,1330,1540,1690,1790,1860,1920,1920,1960,1980,2020,2020,2020,2020,-2500,-2500,-2500,-2440,-2420,-2420,-2380,-2300,-2250,-2180,-2000,-1800,-1540,-1150,-690,0,690,1150,1540,1800,2000,2180,2250,2300,2380,2420,2420,2440,2500,2500,2500],31,5)  InternalRulePriority=Speed  RndMeth=Simplest  InputSameDT=on
  Bus Selector : BusSelector  OutputSignals=SensorBus.Read_ay_m/s²,Vehicle_velocity_mps,SensorBus.Read_Vhcl_YawRate,SensorBus.Read_ax_m/s²,SensorBus.Read_Mean_Steering_Angle_Wheels,SensorBus.Read_Steering_angle_rad
  Memory : Memory  X0=0.001
  Memory1 : Memory  X0=0.001
  Mu_ DroogWegdek : Constant  Value=mu_max
  PI_CONTROLLER1 : Subsystem
  Post-processor : Subsystem
  Pre-processor : Subsystem
  Scope : Scope  NumInputPorts=2
      settings: YMin=-175~-1.5  YMax=25~1.5  SaveName=ScopeData11
  Signal Specification : SignalSpecification  Dimensions=1
  Signal Specification1 : SignalSpecification  Dimensions=1
  Sum4 : Sum  Inputs=|+-
  Trl : Outport
  Trr : Outport  Port=2
  wires:
  Mu_ DroogWegdek/1 -> Pre-processor/3(mu_max), Post-processor/3(mu_max)
  PI_CONTROLLER1/1(PI_out) -> Post-processor/5(Mz)  "Mz"
  Post-processor/1(Trl) -> Trl/1  "Trl"
  Post-processor/2(Trr) -> Trr/1  "Trr"
  Sum4/1 -> PI_CONTROLLER1/1(YawRate-Error)
  Memory/1 -> Pre-processor/7(alfa_r1), 2-D Lookup Table2/1
  Memory1/1 -> 2-D Lookup Table1/1, Pre-processor/8(alfa_f1)
  Pre-processor/2(alfa_f) -> Memory1/1
  Signal Specification1/1 -> Pre-processor/5(Fy_f)
  Signal Specification/1 -> Pre-processor/6(Fy_r)
  Pre-processor/3(alfa_r) -> Memory/1
  2-D Lookup Table2/1 -> Signal Specification/1
  2-D Lookup Table1/1 -> Signal Specification1/1
  Inputs/1 -> Bus Selector/1
  Tgevraagd/1 -> Post-processor/6(Tgevraagd)
  Bus Selector/6 -> ?  "<Read_Steering_angle_rad>"
  Bus Selector/4 -> Pre-processor/4(a_zwpx), Post-processor/1(ax)  "<Read_ax_m/s²>"
  Bus Selector/1 -> Post-processor/2(ay)  "<Read_ay_m/s²>"
  Bus Selector/2 -> Pre-processor/1(Vzwp), Post-processor/4(Vzwp), PI_CONTROLLER1/2(Vzwp)  "<Vehicle_velocity_mps>"
  Post-processor/4(Wr) -> 2-D Lookup Table2/2  "Wr"
  Pre-processor/1(Yaw_ref) -> Scope/1, Sum4/1  "Yaw_ref"
  Bus Selector/3 -> Scope/2, Sum4/2  "<Read_Vhcl_YawRate>"
  Post-processor/3(Wf) -> 2-D Lookup Table1/2  "Wf"
  Bus Selector/5 -> Pre-processor/2(Stuurhoek)  "<Read_Mean_Steering_Angle_Wheels>"

== system generic_IsaacV3/CarMaker/Vehicle Sensors ==
  Bus Creator : BusCreator  Inputs=19
  Gain : Gain  Gain=1/2
  PreProcessor : Subsystem
  Read_BatteryHV_Current_A : CarMaker4SL/Read CM Dict  xname=PT.BattHV.Current  xsync=off
  Read_Driver_brake_0/1 : CarMaker4SL/Read CM Dict  xname=DM.Brake  xsync=off
  Read_Driver_gas_0/1 : CarMaker4SL/Read CM Dict  xname=DM.Gas  xsync=off
  Read_ElecMotorPowerRL_W : CarMaker4SL/Read CM Dict  xname=PT.Motor.PwrElec  xsync=off
  Read_ElecMotorPowerRR_W : CarMaker4SL/Read CM Dict  xname=PT.Motor1.PwrElec  xsync=off
  Read_SpringLenghtFL_m : CarMaker4SL/Read CM Dict  xname=Car.SpringFL.l  xsync=off
  Read_SpringLenghtFR_m : CarMaker4SL/Read CM Dict  xname=Car.SpringFR.l  xsync=off
  Read_SpringLenghtRL_m : CarMaker4SL/Read CM Dict  xname=Car.SpringRL.l  xsync=off
  Read_SpringLenghtRR_m : CarMaker4SL/Read CM Dict  xname=Car.SpringRR.l  xsync=off
  Read_Steering_angle_rad : CarMaker4SL/Read CM Dict  xname=Steer.WhlAng  xsync=off
  Read_Vhcl_SteerAngleFL : CarMaker4SL/Read CM Dict  xname=Car.SteerAngleFL  xsync=off
  Read_Vhcl_SteerAngleFR : CarMaker4SL/Read CM Dict  xname=Car.SteerAngleFR  xsync=off
  Read_Vhcl_YawRate : CarMaker4SL/Read CM Dict  xname=Vhcl.YawRate  xsync=off
  Read_WheelspeedFL_rad/s : CarMaker4SL/Read CM Dict  xname=Vhcl.FL.rotv  xsync=off
  Read_WheelspeedFR_rad/s : CarMaker4SL/Read CM Dict  xname=Vhcl.FR.rotv  xsync=off
  Read_WheelspeedRL_rad/s : CarMaker4SL/Read CM Dict  xname=Vhcl.RL.rotv  xsync=off
  Read_WheelspeedRR_rad/s : CarMaker4SL/Read CM Dict  xname=Vhcl.RR.rotv  xsync=off
  Read_Yawacc_rad/s² : CarMaker4SL/Read CM Dict  xname=Vhcl.YawAcc  xsync=off
  Read_ax_m/s² : CarMaker4SL/Read CM Dict  xname=Car.Con.ax_1  xsync=off
  Read_ay_m/s² : CarMaker4SL/Read CM Dict  xname=Car.Con.ay_1  xsync=off
  SensorIn Plots : Subsystem
  Sum : Sum  Inputs=|++
  convert : Gain  Gain=1/1000
  convert1 : Gain  Gain=1/1000
  Sensor inputs : Outport
  wires:
  Read_Steering_angle_rad/1 -> Bus Creator/1  "Read_Steering_angle_rad"
  Read_Driver_gas_0/1/1 -> Bus Creator/2  "Read_Driver_gas_0/1"
  Read_Driver_brake_0/1/1 -> Bus Creator/3  "Read_Driver_brake_0/1"
  Read_Yawacc_rad/s²/1 -> Bus Creator/4  "Read_Yawacc_rad/s²"
  Read_WheelspeedFL_rad/s/1 -> Bus Creator/5  "Read_WheelspeedFL_rad/s"
  Read_WheelspeedFR_rad/s/1 -> Bus Creator/6  "Read_WheelspeedFR_rad/s"
  Read_WheelspeedRL_rad/s/1 -> Bus Creator/7  "Read_WheelspeedRL_rad/s"
  Read_WheelspeedRR_rad/s/1 -> Bus Creator/8  "Read_WheelspeedRR_rad/s"
  Read_ax_m/s²/1 -> Bus Creator/9  "Read_ax_m/s²"
  Read_ay_m/s²/1 -> Bus Creator/10  "Read_ay_m/s²"
  Read_SpringLenghtFL_m/1 -> Bus Creator/11  "Read_SpringLenghtFL_m"
  Read_SpringLenghtFR_m/1 -> Bus Creator/12  "Read_SpringLenghtFR_m"
  Read_SpringLenghtRL_m/1 -> Bus Creator/14  "Read_SpringLenghtRL_m"
  Read_SpringLenghtRR_m/1 -> Bus Creator/13  "Read_SpringLenghtRR_m"
  Bus Creator/1 -> PreProcessor/1(SensorBus)  "SensorBus"
  Read_BatteryHV_Current_A/1 -> Bus Creator/15  "Read_BatteryHV_Current_A"
  Read_ElecMotorPowerRL_W/1 -> convert/1  "Read_ElecMotorPowerRL_W"
  Read_ElecMotorPowerRR_W/1 -> convert1/1  "Read_ElecMotorPowerRR_W"
  convert/1 -> Bus Creator/16  "Read_ElecMotorPowerRL_kW"
  convert1/1 -> Bus Creator/17  "Read_ElecMotorPowerRR_kW"
  PreProcessor/1(SensorBusOut) -> Sensor inputs/1, SensorIn Plots/1(SensorBus)
  Read_Vhcl_YawRate/1 -> Bus Creator/18  "Read_Vhcl_YawRate"
  Read_Vhcl_SteerAngleFL/1 -> Sum/1
  Read_Vhcl_SteerAngleFR/1 -> Sum/2
  Sum/1 -> Gain/1
  Gain/1 -> Bus Creator/19  "Read_Mean_Steering_Angle_Wheels"

== system generic_IsaacV3/CarMaker/VehicleControl ==
  note: <Your model here>
  note: When implementing a vehicle control model,
      | be sure to add '-disablevehiclecontrol' to the command line arguments
      | in the CarMaker Model Configuration block.
      | Otherwise your model will possibly not see the original DrivMan signals
      | on its inputs, but those of a currently activated C-coded vehicle control model instead.
  Sync_In : Inport
  DrivMan.In : Inport  Port=2
  Bus Creator2 : BusCreator  Inputs=2
  CreateBus Vhcl.Misc : Subsystem
  CreateBus Vhcl.Wheel.In : Subsystem
  CreateBus VhclCtrl : Subsystem
  CreateBus VhclCtrl.PT : Subsystem
  CreateBus VhclCtrl.Steering : Subsystem
  Demux2 : Demux  Outputs=2
  VehicleControl : S-Function  FunctionName=CM_Sfun  Parameters='VehicleControl'
  VehicleControlUpd : S-Function  FunctionName=CM_Sfun  Parameters='VehicleControlUpd'
  Sync_Out : Outport
  Vhcl.Model.Source : Outport  Port=2
  VhclCtrl.Steering : Outport  Port=3
  Vhcl.Wheel.In : Outport  Port=4
  Vhcl.Misc : Outport  Port=5
  VhclCtrl.Brake : Outport  Port=6
  VhclCtrl.PT : Outport  Port=7
  wires:
  CreateBus VhclCtrl/1(Out) -> VehicleControlUpd/2
  VehicleControl/2 -> CreateBus VhclCtrl/1(In)
  VehicleControlUpd/2 -> Vhcl.Model.Source/1
  VehicleControlUpd/4 -> CreateBus Vhcl.Wheel.In/1(In1)
  VehicleControlUpd/5 -> CreateBus Vhcl.Misc/1(In1)
  VehicleControlUpd/6 -> Demux2/1
  VehicleControlUpd/7 -> CreateBus VhclCtrl.PT/1(In1)
  VehicleControlUpd/3 -> CreateBus VhclCtrl.Steering/1(In1)
  CreateBus Vhcl.Misc/1(Out1) -> Vhcl.Misc/1
  CreateBus Vhcl.Wheel.In/1(Out1) -> Vhcl.Wheel.In/1
  DrivMan.In/1 -> VehicleControl/2
  VehicleControl/1 -> VehicleControlUpd/1
  Sync_In/1 -> VehicleControl/1
  CreateBus VhclCtrl.PT/1(Out1) -> VhclCtrl.PT/1
  Bus Creator2/1 -> VhclCtrl.Brake/1
  CreateBus VhclCtrl.Steering/1(Out1) -> VhclCtrl.Steering/1
  VehicleControlUpd/1 -> Sync_Out/1
  Demux2/2 -> Bus Creator2/2  "VhclCtrl BrakePark"
  Demux2/1 -> Bus Creator2/1  "VhclCtrl Brake"

== system generic_IsaacV3/CarMaker/E-diff/E-Differential ==
  Accelerating : Inport
  Velocity : Inport  Port=2
  SteeringAngle : Inport  Port=3
  Constant : Constant  Value=MaxSteeringAngle
  Constant1 : Constant  Value=TrackWidth
  Constant2 : Constant  Value=DifferentialFactor
  Constant3 : Constant  Value=TrackLength
  Constant4 : Constant  Value=GearRatio
  Constant5 : Constant  Value=TireRadius
  Differential : MATLAB Function  TreatAsAtomicUnit=on
  DMC1_SpeedRq : Outport
  DMC2_SpeedRq : Outport  Port=2
  wires:
  SteeringAngle/1 -> Differential/2(SteeringAngle)
  Velocity/1 -> Differential/3(Velocity)
  Constant2/1 -> Differential/4(DifferentialFactor)
  Differential/2(MaxSpeedLeft_rpm) -> DMC2_SpeedRq/1  "DMC2_SpeedRq"
  Differential/1(MaxSpeedRight_rpm) -> DMC1_SpeedRq/1  "DMC1_SpeedRq"
  Accelerating/1 -> Differential/1(Accelerating)
  Constant/1 -> Differential/5(MaxSteeringAngle)
  Constant1/1 -> Differential/6(TrackWidth)
  Constant3/1 -> Differential/7(TrackLength)
  Constant4/1 -> Differential/8(GearRatio)
  Constant5/1 -> Differential/9(TireRadius)

== system generic_IsaacV3/CarMaker/IPG Vehicle/Brake ==
  note: <Your model here>
  note: When replacing the entire braking system,
      | be sure to add '-disablebrake' to the command line arguments
      | in the CarMaker Model Configuration block.
  Sync_In : Inport
  Brake.IF.In : Inport  Port=2
  VhclCtrl.Brake : Inport  Port=3
  Brake : S-Function  FunctionName=CM_Sfun  Parameters='Brake'
  BrakeUpd : S-Function  FunctionName=CM_Sfun  Parameters='BrakeUpd'
  BusCreator : BusCreator  Inputs=12
  CreateBus Vhcl.Wheel.PT : Subsystem
  Demux : Demux  Outputs=12
  Sync_Out : Outport
  Vhcl.Wheel.PT : Outport  Port=2
  wires:
  BrakeUpd/1 -> Sync_Out/1
  Brake/1 -> BrakeUpd/1  "Sync"
  Brake.IF.In/1 -> Brake/2
  VhclCtrl.Brake/1 -> Brake/3
  Brake/2 -> Demux/1
  BusCreator/1 -> BrakeUpd/2
  Sync_In/1 -> Brake/1
  Demux/12 -> BusCreator/12  "Brake IF Trq_Reg_trg RR"
  Demux/11 -> BusCreator/11  "Brake IF Trq_Reg_trg RL"
  Demux/10 -> BusCreator/10  "Brake IF Trq_Reg_trg FR"
  Demux/9 -> BusCreator/9  "Brake IF Trq_Reg_trg FL"
  Demux/8 -> BusCreator/8  "Brake IF Trq_PB RR"
  Demux/7 -> BusCreator/7  "Brake IF Trq_PB RL"
  Demux/6 -> BusCreator/6  "Brake IF Trq_PB FR"
  Demux/5 -> BusCreator/5  "Brake IF Trq_PB FL"
  Demux/4 -> BusCreator/4  "Brake IF Trq_WB RR"
  Demux/3 -> BusCreator/3  "Brake IF Trq_WB RL"
  Demux/2 -> BusCreator/2  "Brake IF Trq_WB FR"
  Demux/1 -> BusCreator/1  "Brake IF Trq_WB FL"
  BrakeUpd/2 -> CreateBus Vhcl.Wheel.PT/1(In)
  CreateBus Vhcl.Wheel.PT/1(Out) -> Vhcl.Wheel.PT/1

== system generic_IsaacV3/CarMaker/IPG Vehicle/CarAndTrailer ==
  Sync_In : Inport
  VhclCtrl.Steering : Inport  Port=2
  Vhcl.Wheel.In : Inport  Port=3
  Vhcl.Misc : Inport  Port=4
  CarAndTrailerUpd : Subsystem
  Forces : Subsystem
  Ground : Ground
  Kinematics : Subsystem
  Kinetics : Subsystem
  Steering : Subsystem
  Terminator : Terminator
  Terminator1 : Terminator
  Trailer : Subsystem
  Sync_Out : Outport
  Brake.IF.In : Outport  Port=2
  wires:
  Trailer/9(Car.Hitch.FrcTrq) -> CarAndTrailerUpd/9(Car.Hitch.FrcTrq)
  Trailer/8(Vhcl.Wheel.RR) -> CarAndTrailerUpd/8(Vhcl.Wheel.RR)
  Trailer/7(Vhcl.Wheel.RL) -> CarAndTrailerUpd/7(Vhcl.Wheel.RL)
  Trailer/6(Vhcl.Wheel.FR) -> CarAndTrailerUpd/6(Vhcl.Wheel.FR)
  Trailer/5(Vhcl.Wheel.FL) -> CarAndTrailerUpd/5(Vhcl.Wheel.FL)
  Trailer/4(Vhcl.PoI) -> CarAndTrailerUpd/4(Vhcl.PoI)
  Trailer/3(Vhcl.Motion) -> CarAndTrailerUpd/3(Vhcl.Motion)
  Trailer/2(Vhcl.Steering) -> CarAndTrailerUpd/2(Vhcl.Steering)
  Trailer/1(Sync_Out) -> CarAndTrailerUpd/1(Sync_In)
  CarAndTrailerUpd/2(Brake.IF.In) -> Brake.IF.In/1
  CarAndTrailerUpd/1(Sync_Out) -> Sync_Out/1
  Vhcl.Misc/1 -> Terminator1/1
  Vhcl.Wheel.In/1 -> Terminator/1
  Kinetics/6(WheelCarrier.Misc) -> Trailer/6(WheelCarrier.Misc)
  Kinetics/5(Car.Trq_T2W) -> Trailer/5(Car.Trq_T2W)
  Steering/2(Steer.IF) -> Kinematics/2(Steer.IF)
  Kinetics/4(Car.Fr1) -> Trailer/4(Car.Fr1)
  Kinetics/3(Car.Hitch) -> Trailer/3(Car.Hitch)
  Kinetics/2(Trailer.Load) -> Trailer/2(Trailer.Load)
  VhclCtrl.Steering/1 -> Steering/2(VhclCtrl.Steering)
  Sync_In/1 -> Steering/1(Sync_In)
  Steering/1(Sync_Out) -> Kinematics/1(Sync_In)
  Kinetics/1(Sync_Out) -> Trailer/1(Sync_In)
  Ground/1 -> CarAndTrailerUpd/10(Vhcl.Fr1A)
  Forces/11(FStabi) -> Kinetics/11(FStabi)
  Forces/10(FDamp) -> Kinetics/10(FDamp)
  Forces/9(FSpring) -> Kinetics/9(FSpring)
  Forces/8(TireRR_Out) -> Kinetics/8(TireRR.Out)
  Forces/7(TireRL_Out) -> Kinetics/7(TireRL.Out)
  Forces/6(TireFR_Out) -> Kinetics/6(TireFR.Out)
  Forces/5(TireFL_Out) -> Kinetics/5(TireFL.Out)
  Forces/4(Car.Load) -> Kinetics/4(Car.Load)
  Forces/2(Car.Virtual) -> Kinetics/2(Car.Virtual)
  Kinematics/6(lSpring) -> Forces/6(lSpring)
  Kinematics/7(vDamp) -> Forces/7(vDamp)
  Forces/3(Car.Aero) -> Kinetics/3(Car.Aero)
  Forces/1(Sync_Out) -> Kinetics/1(Sync_In)
  Kinematics/5(TireRR_In) -> Forces/5(TireRR_In)
  Kinematics/4(TireRL_In) -> Forces/4(TireRL_In)
  Kinematics/3(TireFR_In) -> Forces/3(TireFR_In)
  Kinematics/2(TireFL_In) -> Forces/2(TireFL_In)
  Kinematics/1(Sync_Out) -> Forces/1(Sync_In)
  Kinematics/8(lStabi) -> Forces/8(lStabi)
  Forces/12(FBuf) -> Kinetics/12(FBuf)
  Kinematics/9(lBuf) -> Forces/9(lBuf)

== system generic_IsaacV3/CarMaker/IPG Vehicle/PowerTrain ==
  note: When replacing the entire powertrain,
      | be sure to add '-disablepowertrain' to the command line arguments
      | in the CarMaker Model Configuration block.
  note: <Your model here>
  Sync_In : Inport
  Vhcl.Wheel.PT : Inport  Port=2
  VhclCtrl.PT : Inport  Port=3
  BusCreator : BusCreator  Inputs=40
  Demux : Demux  Outputs=40
  PowerTrain : S-Function  FunctionName=CM_Sfun  Parameters='PowerTrain'
  PowerTrainUpd : S-Function  FunctionName=CM_Sfun  Parameters='PowerTrainUpd'
  Sync_Out : Outport
  wires:
  Sync_In/1 -> PowerTrain/1
  PowerTrain/2 -> Demux/1
  PowerTrainUpd/1 -> Sync_Out/1
  PowerTrain/1 -> PowerTrainUpd/1  "Sync"
  BusCreator/1 -> PowerTrainUpd/2
  Demux/1 -> BusCreator/1  "PT IF Ignition"
  Demux/2 -> BusCreator/2  "PT IF OperationState"
  Demux/3 -> BusCreator/3  "PT IF OperationError"
  Demux/4 -> BusCreator/4  "PT IF GearNo"
  Demux/5 -> BusCreator/5  "PT IF Engine_rotv"
  Demux/6 -> BusCreator/6  "PT IF Engine_Trq (EngineControl)"
  Demux/8 -> BusCreator/8  "PT IF Trq_Supp2Bdy1 y"
  Demux/9 -> BusCreator/9  "PT IF Trq_Supp2Bdy1 z"
  Demux/10 -> BusCreator/10  "PT IF Trq_Supp2BdyEng x"
  Demux/11 -> BusCreator/11  "PT IF Trq_Supp2BdyEng y"
  Demux/12 -> BusCreator/12  "PT IF DL_iDiff_mean"
  Demux/13 -> BusCreator/13  "PT IF WFL rot"
  Demux/14 -> BusCreator/14  "PT IF WFL rotv"
  Demux/15 -> BusCreator/15  "PT IF WFL Trq_B2W"
  Demux/17 -> BusCreator/17  "PT IF WFL Trq_Supp2WC"
  Demux/18 -> BusCreator/18  "PT IF WFL Trq_BrakeReg"
  Demux/19 -> BusCreator/19  "PT IF WFL Trq_BrakeReg_max"
  Demux/20 -> BusCreator/20  "PT IF WFR rot"
  Demux/25 -> BusCreator/25  "PT IF WFR Trq_BrakeReg"
  Demux/26 -> BusCreator/26  "PT IF WFR Trq_BrakeReg_max"
  Demux/27 -> BusCreator/27  "PT IF WRL rot"
  Demux/28 -> BusCreator/28  "PT IF WRL rotv"
  Demux/31 -> BusCreator/31  "PT IF WRL Trq_Supp2WC"
  Demux/32 -> BusCreator/32  "PT IF WRL Trq_BrakeReg"
  Demux/33 -> BusCreator/33  "PT IF WRL Trq_BrakeReg_max"
  Demux/34 -> BusCreator/34  "PT IF WRR rot"
  Demux/35 -> BusCreator/35  "PT IF WRR rotv"
  Demux/36 -> BusCreator/36  "PT IF WRR Trq_B2W"
  Demux/37 -> BusCreator/37  "PT IF WRR Trq_Drive"
  Demux/39 -> BusCreator/39  "PT IF WRR Trq_BrakeReg"
  Demux/40 -> BusCreator/40  "PT IF WRR Trq_BrakeReg_max"
  VhclCtrl.PT/1 -> PowerTrain/3
  Vhcl.Wheel.PT/1 -> PowerTrain/2
  Demux/29 -> BusCreator/29  "PT IF WRL Trq_B2W"
  Demux/7 -> BusCreator/7  "PT IF Trq_Supp2Bdy1 x"
  Demux/16 -> BusCreator/16  "PT IF WFL Trq_Drive"
  Demux/21 -> BusCreator/21  "PT IF WFR rotv"
  Demux/22 -> BusCreator/22  "PT IF WFR Trq_B2W"
  Demux/23 -> BusCreator/23  "PT IF WFR Trq_Drive"
  Demux/24 -> BusCreator/24  "PT IF WFR Trq_Supp2WC"
  Demux/30 -> BusCreator/30  "PT IF WRL Trq_Drive"
  Demux/38 -> BusCreator/38  "PT IF WRR Trq_Supp2WC"

== system generic_IsaacV3/CarMaker/SignalOut/CreateBus PTC ClutchOut ==
  In : Inport
  BusCreator : BusCreator  Inputs=3
  Demux : Demux  Outputs=3
  Out : Outport
  wires:
  In/1 -> Demux/1
  BusCreator/1 -> Out/1
  Demux/1 -> BusCreator/1  "PTC ClutchOut Pos"
  Demux/2 -> BusCreator/2  "PTC ClutchOut rotv_out_trg"
  Demux/3 -> BusCreator/3  "PTC ClutchOut Trq_out_trg"

== system generic_IsaacV3/CarMaker/SignalOut/CreateBus PTC EngineOut ==
  In : Inport
  BusCreator : BusCreator  Inputs=5
  Demux : Demux  Outputs=5
  Out : Outport
  wires:
  In/1 -> Demux/1
  BusCreator/1 -> Out/1
  Demux/1 -> BusCreator/1  "PTC EngineOut set_ISC"
  Demux/2 -> BusCreator/2  "PTC EngineOut FuelCutOff"
  Demux/3 -> BusCreator/3  "PTC EngineOut Load"
  Demux/4 -> BusCreator/4  "PTC EngineOut Trq_trg"
  Demux/5 -> BusCreator/5  "PTC EngineOut rotv_trg"

== system generic_IsaacV3/CarMaker/SignalOut/CreateBus PTC GearBoxM_Out0 ==
  In : Inport
  BusCreator : BusCreator  Inputs=7
  Demux : Demux  Outputs=7
  Out : Outport
  wires:
  In/1 -> Demux/1
  BusCreator/1 -> Out/1
  Demux/1 -> BusCreator/1  "PTC GearBoxM_Out0 GearNoTrg"
  Demux/2 -> BusCreator/2  "PTC GearBoxM_Out0 set_ParkBrake"
  Demux/3 -> BusCreator/3  "PTC GearBoxM_Out0 rotv_in_trg"
  Demux/4 -> BusCreator/4  "PTC GearBoxM_Out0 Trq_out_trg"
  Demux/5 -> BusCreator/5  "PTC GearBoxM_Out0 Clutch Pos"
  Demux/6 -> BusCreator/6  "PTC GearBoxM_Out0 Clutch rotv_out_trg"
  Demux/7 -> BusCreator/7  "PTC GearBoxM_Out0 Clutch Trq_out_trg"

== system generic_IsaacV3/CarMaker/SignalOut/CreateBus PTC GearBoxM_Out1 ==
  In : Inport
  BusCreator : BusCreator  Inputs=7
  Demux : Demux  Outputs=7
  Out : Outport
  wires:
  In/1 -> Demux/1
  BusCreator/1 -> Out/1
  Demux/1 -> BusCreator/1  "PTC GearBoxM_Out1 GearNoTrg"
  Demux/2 -> BusCreator/2  "PTC GearBoxM_Out1 set_ParkBrake"
  Demux/3 -> BusCreator/3  "PTC GearBoxM_Out1 rotv_in_trg"
  Demux/4 -> BusCreator/4  "PTC GearBoxM_Out1 Trq_out_trg"
  Demux/5 -> BusCreator/5  "PTC GearBoxM_Out1 Clutch Pos"
  Demux/6 -> BusCreator/6  "PTC GearBoxM_Out1 Clutch rotv_out_trg"
  Demux/7 -> BusCreator/7  "PTC GearBoxM_Out1 Clutch Trq_out_trg"

== system generic_IsaacV3/CarMaker/SignalOut/CreateBus PTC GearBoxM_Out2 ==
  In : Inport
  BusCreator : BusCreator  Inputs=7
  Demux : Demux  Outputs=7
  Out : Outport
  wires:
  In/1 -> Demux/1
  BusCreator/1 -> Out/1
  Demux/1 -> BusCreator/1  "PTC GearBoxM_Out2 GearNoTrg"
  Demux/2 -> BusCreator/2  "PTC GearBoxM_Out2 set_ParkBrake"
  Demux/3 -> BusCreator/3  "PTC GearBoxM_Out2 rotv_in_trg"
  Demux/4 -> BusCreator/4  "PTC GearBoxM_Out2 Trq_out_trg"
  Demux/5 -> BusCreator/5  "PTC GearBoxM_Out2 Clutch Pos"
  Demux/6 -> BusCreator/6  "PTC GearBoxM_Out2 Clutch rotv_out_trg"
  Demux/7 -> BusCreator/7  "PTC GearBoxM_Out2 Clutch Trq_out_trg"

== system generic_IsaacV3/CarMaker/SignalOut/CreateBus PTC GearBoxM_Out3 ==
  In : Inport
  BusCreator : BusCreator  Inputs=7
  Demux : Demux  Outputs=7
  Out : Outport
  wires:
  In/1 -> Demux/1
  BusCreator/1 -> Out/1
  Demux/1 -> BusCreator/1  "PTC GearBoxM_Out3 GearNoTrg"
  Demux/2 -> BusCreator/2  "PTC GearBoxM_Out3 set_ParkBrake"
  Demux/3 -> BusCreator/3  "PTC GearBoxM_Out3 rotv_in_trg"
  Demux/4 -> BusCreator/4  "PTC GearBoxM_Out3 Trq_out_trg"
  Demux/5 -> BusCreator/5  "PTC GearBoxM_Out3 Clutch Pos"
  Demux/6 -> BusCreator/6  "PTC GearBoxM_Out3 Clutch rotv_out_trg"
  Demux/7 -> BusCreator/7  "PTC GearBoxM_Out3 Clutch Trq_out_trg"

== system generic_IsaacV3/CarMaker/SignalOut/CreateBus PTC GearBoxOut ==
  In : Inport
  BusCreator : BusCreator  Inputs=7
  Demux : Demux  Outputs=7
  Out : Outport
  wires:
  In/1 -> Demux/1
  BusCreator/1 -> Out/1
  Demux/1 -> BusCreator/1  "PTC GearBoxOut GearNoTrg"
  Demux/2 -> BusCreator/2  "PTC GearBoxOut set_ParkBrake"
  Demux/3 -> BusCreator/3  "PTC GearBoxOut rotv_in_trg"
  Demux/4 -> BusCreator/4  "PTC GearBoxOut Trq_out_trg"
  Demux/5 -> BusCreator/5  "PTC GearBoxOut Clutch Pos"
  Demux/6 -> BusCreator/6  "PTC GearBoxOut Clutch rotv_out_trg"
  Demux/7 -> BusCreator/7  "PTC GearBoxOut Clutch Trq_out_trg"

== system generic_IsaacV3/CarMaker/SignalOut/CreateBus PTC ISGOut ==
  In : Inport
  BusCreator : BusCreator  Inputs=3
  Demux : Demux  Outputs=3
  Out : Outport
  wires:
  In/1 -> Demux/1
  BusCreator/1 -> Out/1
  Demux/1 -> BusCreator/1  "PTC ISGOut Load"
  Demux/2 -> BusCreator/2  "PTC ISGOut Trq_trg"
  Demux/3 -> BusCreator/3  "PTC ISGOut rotv_trg"

== system generic_IsaacV3/CarMaker/SignalOut/CreateBus PTC MiscOut ==
  In : Inport
  BusCreator : BusCreator
  Demux : Demux
  Out : Outport
  wires:
  In/1 -> Demux/1
  BusCreator/1 -> Out/1
  Demux/1 -> BusCreator/1  "PTC_Out OperationState"
  Demux/2 -> BusCreator/2  "PTC_Out OperationError"
  Demux/3 -> BusCreator/3  "PTC_Out StrategyMode"
  Demux/4 -> BusCreator/4  "PTC_Out Ignition"
